simulink model "mechanical_model_wn_input"  (R2019b)
settings: Solver=FixedStepAuto  StartTime=0.0  StopTime=31.6  FixedStep=1e-3  RelTol=1e-3
undefined symbols (not defined in the file or in its folder): symTf1, symTf2
settings Model: Creator=Guido  LastModifiedBy=Guido

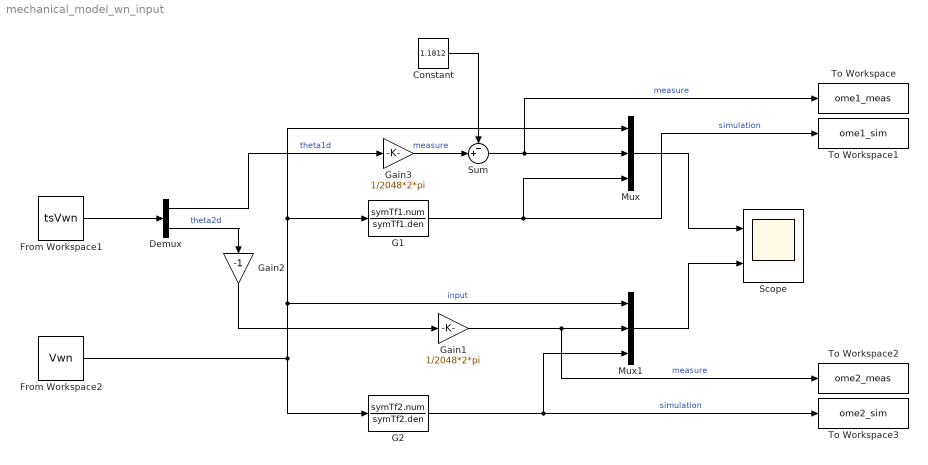
== system mechanical_model_wn_input ==
  Constant : Constant  Value=1.1812
  Demux : Demux  Outputs=2
  From Workspace1 : FromWorkspace  VariableName=tsVwn  SampleTime=0
  From Workspace2 : FromWorkspace  VariableName=Vwn  SampleTime=0
  G1 : TransferFcn  Numerator=symTf1.num  Denominator=symTf1.den
  G2 : TransferFcn  Numerator=symTf2.num  Denominator=symTf2.den
  Gain1 : Gain  Gain=1/2048*2*pi
  Gain2 : Gain  Gain=-1
  Gain3 : Gain  Gain=1/2048*2*pi
  Mux : Mux  Inputs=3
  Mux1 : Mux  Inputs=3
  Scope : Scope  NumInputPorts=2
  Sum : Sum  Inputs=-+|
  To Workspace : ToWorkspace  VariableName=ome1_meas  SaveFormat=Timeseries  SampleTime=-1
  To Workspace1 : ToWorkspace  VariableName=ome1_sim  SaveFormat=Timeseries  SampleTime=-1
  To Workspace2 : ToWorkspace  VariableName=ome2_meas  SaveFormat=Timeseries  SampleTime=-1
  To Workspace3 : ToWorkspace  VariableName=ome2_sim  SaveFormat=Timeseries  SampleTime=-1
  wires:
  Gain1/1 -> To Workspace2/1, Mux1/2  "measure"
  Demux/1 -> Gain3/1  "theta1d"
  Demux/2 -> Gain2/1  "theta2d"
  Mux/1 -> Scope/1
  Mux1/1 -> Scope/2
  G2/1 -> To Workspace3/1, Mux1/3  "simulation"
  Gain2/1 -> Gain1/1
  G1/1 -> Mux/3, To Workspace1/1  "simulation"
  From Workspace1/1 -> Demux/1
  Sum/1 -> To Workspace/1, Mux/2  "measure"
  From Workspace2/1 -> Mux/1, G1/1, Mux1/1, G2/1  "input"
  Gain3/1 -> Sum/2  "measure"
  Constant/1 -> Sum/1
